simulink model "lr6"  (R2022b)
settings: Solver=VariableStepAuto  StartTime=0.0  StopTime=3  MaxStep=0.001  MinStep=0.0001  RelTol=1e-3
undefined symbols (not defined in the file): A, Ad, B, Bd, C, K, L
settings Model: Creator=Dimuss  LastModifiedBy=Dimuss

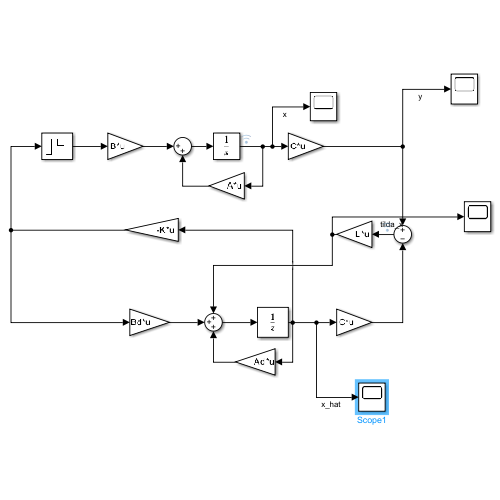
[thumbnail: Simulink's stored preview of the top-level diagram]
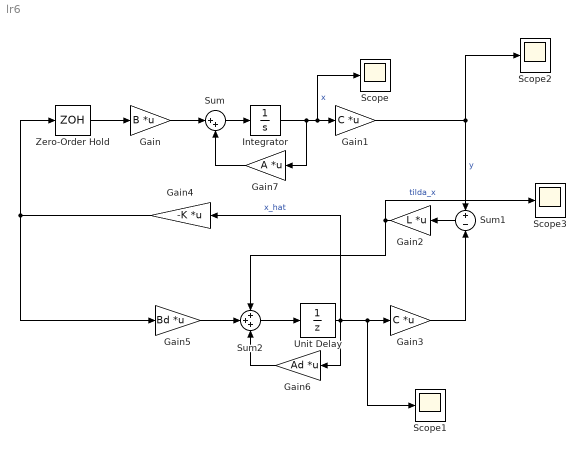
== system lr6 ==
  Gain : Gain  Gain=B  Multiplication=Matrix(K*u)
  Gain1 : Gain  Gain=C  Multiplication=Matrix(K*u)
  Gain2 : Gain  Gain=L  Multiplication=Matrix(K*u)
  Gain3 : Gain  Gain=C  Multiplication=Matrix(K*u)
  Gain4 : Gain  Gain=-K  Multiplication=Matrix(K*u)
  Gain5 : Gain  Gain=Bd  Multiplication=Matrix(K*u)
  Gain6 : Gain  Gain=Ad  Multiplication=Matrix(K*u)
  Gain7 : Gain  Gain=A  Multiplication=Matrix(K*u)
  Integrator : Integrator  InitialCondition=[0.2396;0]
  Scope{,1..3} (4 alike) : Scope
  Sum : Sum  Inputs=|++
  Sum1 : Sum  Inputs=+-
  Sum2 : Sum  Inputs=+++
  Unit Delay : UnitDelay  InitialCondition=[0.2396;0]  SampleTime=-1  HasFrameUpgradeWarning=on
  Zero-Order Hold : ZeroOrderHold  SampleTime=0.4
  wires:
  Zero-Order Hold/1 -> Gain/1
  Gain/1 -> Sum/1
  Sum/1 -> Integrator/1
  Integrator/1 -> Gain7/1, Scope/1, Gain1/1  "x"
  Gain1/1 -> Sum1/1, Scope2/1  "y"
  Sum1/1 -> Gain2/1
  Sum2/1 -> Unit Delay/1
  Unit Delay/1 -> Gain4/1, Gain6/1, Scope1/1, Gain3/1  "x_hat"
  Gain3/1 -> Sum1/2
  Gain2/1 -> Scope3/1, Sum2/1  "tilda_x"
  Gain4/1 -> Gain5/1, Zero-Order Hold/1
  Gain5/1 -> Sum2/2
  Gain6/1 -> Sum2/3
  Gain7/1 -> Sum/2
